simulink model "ACC_speed_change_curve_cs"  (R2016a)
settings: Solver=ode5  SolverMode=SingleTasking  StartTime=0.0  StopTime=inf  FixedStep=1/1000  RelTol=1e-3
PreLoadFcn:
  | mbxruntime.callbacks.PreLoadFcn(bdroot);
  | check_NUTS_defined;
  | 
  | assignin('base',['model_closed_' bdroot],false);addpath('../includes_ACC');
PostLoadFcn:
  | mbxruntime.callbacks.PostLoadFcn(bdroot);
InitFcn:
  | mbxruntime.callbacks.InitFcn(bdroot);
StartFcn:
  | mbxruntime.callbacks.StartFcn(bdroot);
StopFcn:
  | mbxruntime.callbacks.StopFcn(bdroot);
model workspace (MAT data in the model file):
  mbox_table : struct (value not decoded)
  model_closed = 0
  sim_status = 0
undefined symbols (not defined in the file or in its folder): DiscIntNeverNeededParam
undefined symbols (not defined in the file): SteeringColumn, SteeringWheel, WheelL0, WheelL1, WheelR0, WheelR1
libraries: simulink_extras x49, simulink x29, PreScanSimulinkLibrary x24, PreScanUsefulBlocks x2, Solver_SF x1, simulink_need_slupdate x1
(part 17 of 17)

== system ACC_speed_change_curve_cs/Audi_A8_1/ACC_System3/TIS2 ACC action/Stop & Go/Subsystem ==
  In1 : Inport
  In2 : Inport  Port=2
  EGO_Velocity [m/s] : Inport  Port=3
  Abs : Abs
  Abs1 : Abs
  Compare To Constant : simulink/Logic and Bit Operations/Compare To Constant  relop=<=  const=0.1  OutDataTypeStr=uint8  ZeroCross=off
  Compare To Constant1 : simulink/Logic and Bit Operations/Compare To Constant  relop=<=  const=0.1  OutDataTypeStr=uint8  ZeroCross=off
  Logical Operator1 : Logic  AllPortsSameDT=off  OutDataTypeStr=boolean
  Max Brake ON : Constant  Value=BrakeMax * J_xx / Qfac / Rw
  Switch1 : Switch  Criteria=u2 > Threshold
  BrakePres[bar] : Outport
  wires:
  In2/1 -> Switch1/3
  Abs1/1 -> Compare To Constant1/1
  Abs/1 -> Compare To Constant/1
  Switch1/1 -> BrakePres[bar]/1
  Max Brake ON/1 -> Switch1/1
  Logical Operator1/1 -> Switch1/2
  Compare To Constant1/1 -> Logical Operator1/2
  Compare To Constant/1 -> Logical Operator1/1
  EGO_Velocity [m/s]/1 -> Abs1/1
  In1/1 -> Abs/1

== system ACC_speed_change_curve_cs/Audi_A8_1/ACC_System3/TIS2 Bend Road/Hold/If Action Subsystem ==
  In1 : Inport
  Action Port : ActionPort  InitializeStates=reset  PropagateVarSize=During execution  ActionType=then
  Constant : Constant
  Constant1 : Constant  Value=0
  Discrete-Time Integrator : DiscreteIntegrator  gainval=100  InitialConditionSource=external  InitialConditionSetting=State (most efficient)  SampleTime=Tsensor  LimitOutput=on  UpperSaturationLimit=1  LowerSaturationLimit=0  ICPrevOutput=DiscIntNeverNeededParam  ICPrevScaledInput=DiscIntNeverNeededParam
  Gain3 : Gain  Gain=1e6  OutDataTypeStr=double
  Switch : Switch  Criteria=u2 > Threshold
  Out1 : Outport
  wires:
  Constant1/1 -> Switch/3
  Constant/1 -> Switch/1
  Switch/1 -> Discrete-Time Integrator/2
  Discrete-Time Integrator/1 -> Out1/1
  In1/1 -> Switch/2, Gain3/1
  Gain3/1 -> Discrete-Time Integrator/1

== system ACC_speed_change_curve_cs/Audi_A8_1/ACC_System3/TIS2 Bend Road/Hold/If Action Subsystem1 ==
  In1 : Inport
  Action Port : ActionPort  PropagateVarSize=During execution  ActionType=else
  Out1 : Outport
  wires:
  In1/1 -> Out1/1

== system ACC_speed_change_curve_cs/Audi_A8_1/ACC_System3/TIS2 Bend Road/TIS1 HWT Computing/If Action Subsystem ==
  Distance [m] : Inport
  Velocity [m/s] : Inport  Port=2
  Action Port : ActionPort  PropagateVarSize=During execution  ActionType=then
  Product : Product  Inputs=*/  RndMeth=Zero
  HWT [s] : Outport
  wires:
  Product/1 -> HWT [s]/1
  Velocity [m/s]/1 -> Product/2
  Distance [m]/1 -> Product/1

== system ACC_speed_change_curve_cs/Audi_A8_1/ACC_System3/TIS2 Bend Road/TIS1 HWT Computing/If Action Subsystem1 ==
  Action Port : ActionPort  PropagateVarSize=During execution  ActionType=else
  Constant : Constant  Value=inf
  Out1 : Outport  InitialOutput=0
  wires:
  Constant/1 -> Out1/1

== system ACC_speed_change_curve_cs/Audi_A8_1/ACC_System3/TIS2 Straight Road/Hold/If Action Subsystem ==
  In1 : Inport
  Action Port : ActionPort  InitializeStates=reset  PropagateVarSize=During execution  ActionType=then
  Constant : Constant
  Constant1 : Constant  Value=0
  Discrete-Time Integrator : DiscreteIntegrator  gainval=100  InitialConditionSource=external  InitialConditionSetting=State (most efficient)  SampleTime=Tsensor  LimitOutput=on  UpperSaturationLimit=1  LowerSaturationLimit=0  ICPrevOutput=DiscIntNeverNeededParam  ICPrevScaledInput=DiscIntNeverNeededParam
  Gain3 : Gain  Gain=1e6  OutDataTypeStr=double
  Switch : Switch  Criteria=u2 > Threshold
  Out1 : Outport
  wires:
  Constant1/1 -> Switch/3
  Constant/1 -> Switch/1
  Switch/1 -> Discrete-Time Integrator/2
  Discrete-Time Integrator/1 -> Out1/1
  In1/1 -> Switch/2, Gain3/1
  Gain3/1 -> Discrete-Time Integrator/1

== system ACC_speed_change_curve_cs/Audi_A8_1/ACC_System3/TIS2 Straight Road/Hold/If Action Subsystem1 ==
  In1 : Inport
  Action Port : ActionPort  PropagateVarSize=During execution  ActionType=else
  Out1 : Outport
  wires:
  In1/1 -> Out1/1

== system ACC_speed_change_curve_cs/Audi_A8_1/ACC_System3/TIS2 Straight Road/TIS2 HWT Computing/If Action Subsystem ==
  Distance [m] : Inport
  Velocity [m/s] : Inport  Port=2
  Action Port : ActionPort  PropagateVarSize=During execution  ActionType=then
  Product : Product  Inputs=*/  RndMeth=Zero
  HWT [s] : Outport
  wires:
  Product/1 -> HWT [s]/1
  Velocity [m/s]/1 -> Product/2
  Distance [m]/1 -> Product/1

== system ACC_speed_change_curve_cs/Audi_A8_1/ACC_System3/TIS2 Straight Road/TIS2 HWT Computing/If Action Subsystem1 ==
  HWT demanded [s] : Inport
  Action Port : ActionPort  PropagateVarSize=During execution  ActionType=else
  Gain : Gain  Gain=2*ones(TISdet(2),1)
  Out1 : Outport
  wires:
  HWT demanded [s]/1 -> Gain/1
  Gain/1 -> Out1/1

== system ACC_speed_change_curve_cs/Audi_A8_1/ACC_System3/TIS2 Straight Road/TIS2 HWT Computing2/If Action Subsystem ==
  Distance [m] : Inport
  Velocity [m/s] : Inport  Port=2
  Action Port : ActionPort  PropagateVarSize=During execution  ActionType=then
  Product : Product  Inputs=*/  RndMeth=Zero
  HWT [s] : Outport
  wires:
  Product/1 -> HWT [s]/1
  Velocity [m/s]/1 -> Product/2
  Distance [m]/1 -> Product/1

== system ACC_speed_change_curve_cs/Audi_A8_1/ACC_System3/TIS2 Straight Road/TIS2 HWT Computing2/If Action Subsystem1 ==
  Action Port : ActionPort  PropagateVarSize=During execution  ActionType=else
  Constant : Constant  Value=inf
  Out1 : Outport  InitialOutput=0
  wires:
  Constant/1 -> Out1/1

== system ACC_speed_change_curve_cs/Audi_A8_1/Trajectories/Traj2State1/Traj2State2/MuxState ==
  x [m] : Inport
  y [m] : Inport  Port=2
  z [m] : Inport  Port=3
  dx [m/s] : Inport  Port=4
  dy [m/s] : Inport  Port=5
  dz [m/s] : Inport  Port=6
  R [rad] : Inport  Port=7
  P [rad] : Inport  Port=8
  Y [rad] : Inport  Port=9
  Mux : Mux  Inputs=9
  state : Outport
  wires:
  z [m]/1 -> Mux/3
  y [m]/1 -> Mux/2
  x [m]/1 -> Mux/1
  Y [rad]/1 -> Mux/9
  P [rad]/1 -> Mux/8
  R [rad]/1 -> Mux/7
  dz [m/s]/1 -> Mux/6
  dy [m/s]/1 -> Mux/5
  dx [m/s]/1 -> Mux/4
  Mux/1 -> state/1

== system ACC_speed_change_curve_cs/Audi_A8_1/Trajectories/Traj2State1/Traj2State2/Traj2MuxState_Ext ==
  Traj : Inport
  Terminator{1..9} (9 alike) : Terminator
  demux : Subsystem
  x [m] : Outport
  y [m] : Outport  Port=2
  z [m] : Outport  Port=3
  dx [m/s] : Outport  Port=4
  dy [m/s] : Outport  Port=5
  dz [m/s] : Outport  Port=6
  R [rad] : Outport  Port=7
  P [rad] : Outport  Port=8
  Y [rad] : Outport  Port=9
  wires:
  demux/9(Y) -> Y [rad]/1
  demux/7(R) -> R [rad]/1
  demux/5(vely) -> dy [m/s]/1
  demux/4(velx) -> dx [m/s]/1
  demux/10(velR) -> Terminator4/1
  demux/11(velP) -> Terminator5/1
  demux/12(velY) -> Terminator1/1
  demux/13(accx) -> Terminator8/1
  demux/14(accy) -> Terminator9/1
  demux/15(accz) -> Terminator7/1
  demux/18(accY) -> Terminator2/1
  demux/16(accR) -> Terminator3/1
  demux/17(accP) -> Terminator6/1
  demux/3(z) -> z [m]/1
  Traj/1 -> demux/1(traj)
  demux/6(velz) -> dz [m/s]/1
  demux/1(x) -> x [m]/1
  demux/2(y) -> y [m]/1
  demux/8(P) -> P [rad]/1

== system ACC_speed_change_curve_cs/BMW_X5_1/Trajectories/Traj2State1/Traj2State2/MuxState ==
  x [m] : Inport
  y [m] : Inport  Port=2
  z [m] : Inport  Port=3
  dx [m/s] : Inport  Port=4
  dy [m/s] : Inport  Port=5
  dz [m/s] : Inport  Port=6
  R [rad] : Inport  Port=7
  P [rad] : Inport  Port=8
  Y [rad] : Inport  Port=9
  Mux : Mux  Inputs=9
  state : Outport
  wires:
  z [m]/1 -> Mux/3
  y [m]/1 -> Mux/2
  x [m]/1 -> Mux/1
  Y [rad]/1 -> Mux/9
  P [rad]/1 -> Mux/8
  R [rad]/1 -> Mux/7
  dz [m/s]/1 -> Mux/6
  dy [m/s]/1 -> Mux/5
  dx [m/s]/1 -> Mux/4
  Mux/1 -> state/1

== system ACC_speed_change_curve_cs/BMW_X5_1/Trajectories/Traj2State1/Traj2State2/Traj2MuxState_Ext ==
  Traj : Inport
  Terminator{1..9} (9 alike) : Terminator
  demux : Subsystem
  x [m] : Outport
  y [m] : Outport  Port=2
  z [m] : Outport  Port=3
  dx [m/s] : Outport  Port=4
  dy [m/s] : Outport  Port=5
  dz [m/s] : Outport  Port=6
  R [rad] : Outport  Port=7
  P [rad] : Outport  Port=8
  Y [rad] : Outport  Port=9
  wires:
  demux/9(Y) -> Y [rad]/1
  demux/7(R) -> R [rad]/1
  demux/5(vely) -> dy [m/s]/1
  demux/4(velx) -> dx [m/s]/1
  demux/10(velR) -> Terminator4/1
  demux/11(velP) -> Terminator5/1
  demux/12(velY) -> Terminator1/1
  demux/13(accx) -> Terminator8/1
  demux/14(accy) -> Terminator9/1
  demux/15(accz) -> Terminator7/1
  demux/18(accY) -> Terminator2/1
  demux/16(accR) -> Terminator3/1
  demux/17(accP) -> Terminator6/1
  demux/3(z) -> z [m]/1
  Traj/1 -> demux/1(traj)
  demux/6(velz) -> dz [m/s]/1
  demux/1(x) -> x [m]/1
  demux/2(y) -> y [m]/1
  demux/8(P) -> P [rad]/1

== system ACC_speed_change_curve_cs/Toyota_Previa_1/Trajectories/Traj2State1/Traj2State2/MuxState ==
  x [m] : Inport
  y [m] : Inport  Port=2
  z [m] : Inport  Port=3
  dx [m/s] : Inport  Port=4
  dy [m/s] : Inport  Port=5
  dz [m/s] : Inport  Port=6
  R [rad] : Inport  Port=7
  P [rad] : Inport  Port=8
  Y [rad] : Inport  Port=9
  Mux : Mux  Inputs=9
  state : Outport
  wires:
  z [m]/1 -> Mux/3
  y [m]/1 -> Mux/2
  x [m]/1 -> Mux/1
  Y [rad]/1 -> Mux/9
  P [rad]/1 -> Mux/8
  R [rad]/1 -> Mux/7
  dz [m/s]/1 -> Mux/6
  dy [m/s]/1 -> Mux/5
  dx [m/s]/1 -> Mux/4
  Mux/1 -> state/1

== system ACC_speed_change_curve_cs/Toyota_Previa_1/Trajectories/Traj2State1/Traj2State2/Traj2MuxState_Ext ==
  Traj : Inport
  Terminator{1..9} (9 alike) : Terminator
  demux : Subsystem
  x [m] : Outport
  y [m] : Outport  Port=2
  z [m] : Outport  Port=3
  dx [m/s] : Outport  Port=4
  dy [m/s] : Outport  Port=5
  dz [m/s] : Outport  Port=6
  R [rad] : Outport  Port=7
  P [rad] : Outport  Port=8
  Y [rad] : Outport  Port=9
  wires:
  demux/9(Y) -> Y [rad]/1
  demux/7(R) -> R [rad]/1
  demux/5(vely) -> dy [m/s]/1
  demux/4(velx) -> dx [m/s]/1
  demux/10(velR) -> Terminator4/1
  demux/11(velP) -> Terminator5/1
  demux/12(velY) -> Terminator1/1
  demux/13(accx) -> Terminator8/1
  demux/14(accy) -> Terminator9/1
  demux/15(accz) -> Terminator7/1
  demux/18(accY) -> Terminator2/1
  demux/16(accR) -> Terminator3/1
  demux/17(accP) -> Terminator6/1
  demux/3(z) -> z [m]/1
  Traj/1 -> demux/1(traj)
  demux/6(velz) -> dz [m/s]/1
  demux/1(x) -> x [m]/1
  demux/2(y) -> y [m]/1
  demux/8(P) -> P [rad]/1

== system ACC_speed_change_curve_cs/Toyota_Yaris_1/Trajectories/Traj2State1/Traj2State2/MuxState ==
  x [m] : Inport
  y [m] : Inport  Port=2
  z [m] : Inport  Port=3
  dx [m/s] : Inport  Port=4
  dy [m/s] : Inport  Port=5
  dz [m/s] : Inport  Port=6
  R [rad] : Inport  Port=7
  P [rad] : Inport  Port=8
  Y [rad] : Inport  Port=9
  Mux : Mux  Inputs=9
  state : Outport
  wires:
  z [m]/1 -> Mux/3
  y [m]/1 -> Mux/2
  x [m]/1 -> Mux/1
  Y [rad]/1 -> Mux/9
  P [rad]/1 -> Mux/8
  R [rad]/1 -> Mux/7
  dz [m/s]/1 -> Mux/6
  dy [m/s]/1 -> Mux/5
  dx [m/s]/1 -> Mux/4
  Mux/1 -> state/1

== system ACC_speed_change_curve_cs/Toyota_Yaris_1/Trajectories/Traj2State1/Traj2State2/Traj2MuxState_Ext ==
  Traj : Inport
  Terminator{1..9} (9 alike) : Terminator
  demux : Subsystem
  x [m] : Outport
  y [m] : Outport  Port=2
  z [m] : Outport  Port=3
  dx [m/s] : Outport  Port=4
  dy [m/s] : Outport  Port=5
  dz [m/s] : Outport  Port=6
  R [rad] : Outport  Port=7
  P [rad] : Outport  Port=8
  Y [rad] : Outport  Port=9
  wires:
  demux/9(Y) -> Y [rad]/1
  demux/7(R) -> R [rad]/1
  demux/5(vely) -> dy [m/s]/1
  demux/4(velx) -> dx [m/s]/1
  demux/10(velR) -> Terminator4/1
  demux/11(velP) -> Terminator5/1
  demux/12(velY) -> Terminator1/1
  demux/13(accx) -> Terminator8/1
  demux/14(accy) -> Terminator9/1
  demux/15(accz) -> Terminator7/1
  demux/18(accY) -> Terminator2/1
  demux/16(accR) -> Terminator3/1
  demux/17(accP) -> Terminator6/1
  demux/3(z) -> z [m]/1
  Traj/1 -> demux/1(traj)
  demux/6(velz) -> dz [m/s]/1
  demux/1(x) -> x [m]/1
  demux/2(y) -> y [m]/1
  demux/8(P) -> P [rad]/1

== system ACC_speed_change_curve_cs/Audi_A8_1/ACC_System3/TIS1 ACC action/If Action Subsystem/If Action Subsystem/Subsystem ==
  e : Inport
  Difference : simulink/Discrete/Difference  ICPrevInput=0.0  InputProcessing=Inherited  OutMin=[]  OutMax=[]  OutDataType=sfix(16)  OutScaling=2^-10  DoSatur=off
  Discrete-Time Integrator : DiscreteIntegrator  SampleTime=Tsensor  ICPrevOutput=DiscIntNeverNeededParam  ICPrevScaledInput=DiscIntNeverNeededParam
  Gain : Gain  Gain=100
  Gain1 : Gain  Gain=0.5
  Gain2 : Gain  Gain=3.065*0.01
  Sum : Sum  Inputs=+++
  out : Outport
  wires:
  Sum/1 -> out/1
  Difference/1 -> Sum/3
  Discrete-Time Integrator/1 -> Sum/2
  Gain/1 -> Sum/1
  Gain2/1 -> Difference/1
  Gain1/1 -> Discrete-Time Integrator/1
  e/1 -> Gain2/1, Gain/1, Gain1/1

== system ACC_speed_change_curve_cs/Audi_A8_1/ACC_System3/TIS1 ACC action/If Action Subsystem/If Action Subsystem1/If Action Subsystem ==
  rd : Inport
  e [m] : Inport  Port=2
  Action Port : ActionPort  PropagateVarSize=During execution  ActionType=then
  Abs : Abs
  Constant : Constant  Value=0
  Divide : Product  Inputs=*/
  Gain : Gain  Gain=0.5
  Math Function : Math  Operator=square  SaturateOnIntegerOverflow=on
  Saturation1 : Saturate  UpperLimit=inf  LowerLimit=0.02
  deceleration_[m/s2] : Outport  InitialOutput=0
  throttle : Outport  Port=2  InitialOutput=0
  wires:
  Constant/1 -> throttle/1
  Gain/1 -> deceleration_[m/s2]/1
  e [m]/1 -> Abs/1
  Saturation1/1 -> Divide/2
  Abs/1 -> Saturation1/1
  Math Function/1 -> Divide/1
  Divide/1 -> Gain/1
  rd/1 -> Math Function/1

== system ACC_speed_change_curve_cs/Audi_A8_1/ACC_System3/TIS1 ACC action/If Action Subsystem/If Action Subsystem1/If Action Subsystem1 ==
  rd : Inport
  e [m] : Inport  Port=2
  EGO_distance[m] : Inport  Port=3
  HWT_dem : Inport  Port=4
  Vp : Inport  Port=5
  e_acc : Inport  Port=6
  th_in : Inport  Port=7
  Action Port : ActionPort  PropagateVarSize=During execution  ActionType=else
  Add : Sum  Inputs=+-
  If : If  SampleTime=Tsensor
  If Action Subsystem : Subsystem  TreatAsAtomicUnit=on
  If Action Subsystem1 : Subsystem  TreatAsAtomicUnit=on
  Merge : Merge
  Merge1 : Merge
  Product : Product  RndMeth=Zero
  Vp1 : InportShadow  Port=5
  throttle : Outport  InitialOutput=0
  brake : Outport  Port=2  InitialOutput=0
  wires:
  th_in/1 -> If Action Subsystem/2(th_in)
  e_acc/1 -> If Action Subsystem/1(e)
  If Action Subsystem/2(throttle) -> Merge/1
  If Action Subsystem/1(brake) -> Merge1/1
  Merge/1 -> throttle/1
  Merge1/1 -> brake/1
  If Action Subsystem1/1(throttle) -> Merge/2
  If Action Subsystem1/2(brake) -> Merge1/2
  Vp/1 -> If Action Subsystem1/1(Vp)
  e [m]/1 -> If Action Subsystem1/3(e [m])
  rd/1 -> If Action Subsystem1/2(rd)
  If/2 -> If Action Subsystem1/Action
  If/1 -> If Action Subsystem/Action
  Add/1 -> If/1
  Product/1 -> Add/2
  EGO_distance[m]/1 -> Add/1
  Vp1/1 -> Product/2
  HWT_dem/1 -> Product/1

== system ACC_speed_change_curve_cs/Audi_A8_1/ACC_System3/TIS1 ACC action/If Action Subsystem1/If Action Subsystem1/If Action Subsystem ==
  Action Port : ActionPort  PropagateVarSize=During execution  ActionType=then
  Constant : Constant  Value=0
  Constant1 : Constant  Value=BrakeMax
  dec : Outport  InitialOutput=0
  throttle : Outport  Port=2  InitialOutput=0
  wires:
  Constant1/1 -> dec/1
  Constant/1 -> throttle/1

== system ACC_speed_change_curve_cs/Audi_A8_1/ACC_System3/TIS1 ACC action/If Action Subsystem1/If Action Subsystem1/If Action Subsystem1 ==
  rd : Inport
  e [m] : Inport  Port=2
  EGO_distance[m] : Inport  Port=3
  HWT_dem : Inport  Port=4
  Vp : Inport  Port=5
  Action Port : ActionPort  PropagateVarSize=During execution  ActionType=else
  Add : Sum  Inputs=+-
  If : If  SampleTime=Tsensor
  If Action Subsystem : Subsystem  TreatAsAtomicUnit=on
  If Action Subsystem1 : Subsystem  TreatAsAtomicUnit=on
  Merge : Merge
  Merge1 : Merge
  Product : Product  RndMeth=Zero
  Vp1 : InportShadow  Port=5
  throttle : Outport  InitialOutput=0
  brake : Outport  Port=2  InitialOutput=0
  wires:
  If Action Subsystem1/1(throttle) -> Merge/2
  If Action Subsystem1/2(brake) -> Merge1/2
  If Action Subsystem/2(throttle) -> Merge/1
  If Action Subsystem/1(brake) -> Merge1/1
  Merge/1 -> throttle/1
  Merge1/1 -> brake/1
  Vp/1 -> If Action Subsystem1/1(Vp)
  e [m]/1 -> If Action Subsystem1/3(e [m])
  rd/1 -> If Action Subsystem1/2(rd)
  If/2 -> If Action Subsystem1/Action
  If/1 -> If Action Subsystem/Action
  Add/1 -> If/1
  Product/1 -> Add/2
  EGO_distance[m]/1 -> Add/1
  Vp1/1 -> Product/2
  HWT_dem/1 -> Product/1

== system ACC_speed_change_curve_cs/Audi_A8_1/ACC_System3/TIS2 ACC action/If Action Subsystem/If Action Subsystem/Subsystem ==
  e : Inport
  Constant : Constant  Value=p
  Constant1 : Constant  Value=i
  Constant2 : Constant  Value=d
  Difference : simulink/Discrete/Difference  ICPrevInput=0.0  InputProcessing=Inherited  OutMin=[]  OutMax=[]  OutDataType=sfix(16)  OutScaling=2^-10  DoSatur=off
  Discrete-Time Integrator : DiscreteIntegrator  SampleTime=-1  ICPrevOutput=DiscIntNeverNeededParam  ICPrevScaledInput=DiscIntNeverNeededParam
  Gain1 : Gain  Gain=0.3
  Gain2 : Gain  Gain=3.065*0.01
  Product : Product
  Product1 : Product
  Product2 : Product
  Sum : Sum  Inputs=+++
  out : Outport
  wires:
  Sum/1 -> out/1
  Difference/1 -> Sum/3
  Discrete-Time Integrator/1 -> Sum/2
  Product/1 -> Sum/1
  Product2/1 -> Difference/1
  Product1/1 -> Discrete-Time Integrator/1
  e/1 -> Product1/2, Product/2, Product2/1
  Constant/1 -> Product/1
  Constant1/1 -> Product1/1
  Constant2/1 -> Product2/2

== system ACC_speed_change_curve_cs/Audi_A8_1/ACC_System3/TIS2 ACC action/If Action Subsystem/If Action Subsystem1/If Action Subsystem ==
  rd : Inport
  e [m] : Inport  Port=2
  Action Port : ActionPort  PropagateVarSize=During execution  ActionType=then
  Abs : Abs
  Constant : Constant  Value=0
  Constant1 : Constant  Value=b
  Divide : Product  Inputs=*/
  Gain : Gain  Gain=0.5
  Math Function : Math  Operator=square  SaturateOnIntegerOverflow=on
  Product : Product
  Saturation1 : Saturate  UpperLimit=inf  LowerLimit=0.02
  deceleration_[m/s2] : Outport  InitialOutput=0
  throttle : Outport  Port=2  InitialOutput=0
  wires:
  Constant/1 -> throttle/1
  Product/1 -> deceleration_[m/s2]/1
  e [m]/1 -> Abs/1
  Saturation1/1 -> Divide/2
  Abs/1 -> Saturation1/1
  Math Function/1 -> Divide/1
  Divide/1 -> Product/2
  rd/1 -> Math Function/1
  Constant1/1 -> Product/1

== system ACC_speed_change_curve_cs/Audi_A8_1/ACC_System3/TIS2 ACC action/If Action Subsystem/If Action Subsystem1/If Action Subsystem1 ==
  rd : Inport
  e [m] : Inport  Port=2
  EGO_distance[m] : Inport  Port=3
  HWT_dem : Inport  Port=4
  Vp : Inport  Port=5
  e_acc : Inport  Port=6
  th_in : Inport  Port=7
  Action Port : ActionPort  PropagateVarSize=During execution  ActionType=else
  Add : Sum  Inputs=+-
  If : If
  If Action Subsystem : Subsystem  TreatAsAtomicUnit=on
  If Action Subsystem1 : Subsystem  TreatAsAtomicUnit=on
  Merge : Merge
  Merge1 : Merge
  Product : Product  RndMeth=Zero
  Vp1 : InportShadow  Port=5
  throttle : Outport  InitialOutput=0
  brake : Outport  Port=2  InitialOutput=0
  wires:
  th_in/1 -> If Action Subsystem/2(th_in)
  e_acc/1 -> If Action Subsystem/1(e)
  If Action Subsystem/2(throttle) -> Merge/1
  If Action Subsystem/1(brake) -> Merge1/1
  Merge/1 -> throttle/1
  Merge1/1 -> brake/1
  If Action Subsystem1/1(throttle) -> Merge/2
  If Action Subsystem1/2(brake) -> Merge1/2
  Vp/1 -> If Action Subsystem1/1(Vp)
  e [m]/1 -> If Action Subsystem1/3(e [m])
  rd/1 -> If Action Subsystem1/2(rd)
  If/2 -> If Action Subsystem1/Action
  If/1 -> If Action Subsystem/Action
  Add/1 -> If/1
  Product/1 -> Add/2
  EGO_distance[m]/1 -> Add/1
  Vp1/1 -> Product/2
  HWT_dem/1 -> Product/1

== system ACC_speed_change_curve_cs/Audi_A8_1/ACC_System3/TIS2 ACC action/If Action Subsystem1/If Action Subsystem1/If Action Subsystem ==
  Action Port : ActionPort  PropagateVarSize=During execution  ActionType=then
  Constant : Constant  Value=0
  Constant1 : Constant  Value=BrakeMax
  dec : Outport  InitialOutput=0
  throttle : Outport  Port=2  InitialOutput=0
  wires:
  Constant1/1 -> dec/1
  Constant/1 -> throttle/1

== system ACC_speed_change_curve_cs/Audi_A8_1/ACC_System3/TIS2 ACC action/If Action Subsystem1/If Action Subsystem1/If Action Subsystem1 ==
  rd : Inport
  e [m] : Inport  Port=2
  EGO_distance[m] : Inport  Port=3
  HWT_dem : Inport  Port=4
  Vp : Inport  Port=5
  Action Port : ActionPort  PropagateVarSize=During execution  ActionType=else
  Add : Sum  Inputs=+-
  If : If
  If Action Subsystem : Subsystem  TreatAsAtomicUnit=on
  If Action Subsystem1 : Subsystem  TreatAsAtomicUnit=on
  Merge : Merge
  Merge1 : Merge
  Product : Product  RndMeth=Zero
  Vp1 : InportShadow  Port=5
  throttle : Outport  InitialOutput=0
  brake : Outport  Port=2  InitialOutput=0
  wires:
  If Action Subsystem/2(throttle) -> Merge/1
  If Action Subsystem/1(brake) -> Merge1/1
  Merge/1 -> throttle/1
  Merge1/1 -> brake/1
  If Action Subsystem1/1(throttle) -> Merge/2
  If Action Subsystem1/2(brake) -> Merge1/2
  Vp/1 -> If Action Subsystem1/1(Vp)
  e [m]/1 -> If Action Subsystem1/3(e [m])
  rd/1 -> If Action Subsystem1/2(rd)
  If/2 -> If Action Subsystem1/Action
  If/1 -> If Action Subsystem/Action
  Add/1 -> If/1
  Product/1 -> Add/2
  EGO_distance[m]/1 -> Add/1
  Vp1/1 -> Product/2
  HWT_dem/1 -> Product/1

== system ACC_speed_change_curve_cs/Audi_A8_1/ACC_System3/TIS2 ACC action/Stop & Go/If Action Subsystem/If Action Subsystem ==
  rd : Inport
  e [m] : Inport  Port=2
  th_in : Inport  Port=3
  dis : Inport  Port=4
  Stand : Inport  Port=5
  Action Port : ActionPort  PropagateVarSize=During execution  ActionType=then
  If : If
  If Action Subsystem : Subsystem  TreatAsAtomicUnit=on
  If Action Subsystem1 : Subsystem  TreatAsAtomicUnit=on
  Merge : Merge
  Merge1 : Merge
  brake : Outport  InitialOutput=0
  throttle : Outport  Port=2  InitialOutput=0
  wires:
  Stand/1 -> If Action Subsystem/4(stand)
  dis/1 -> If Action Subsystem/3(dis)
  th_in/1 -> If Action Subsystem1/2(th_in)
  If Action Subsystem1/2(throttle) -> Merge1/2
  If Action Subsystem1/1(brake) -> Merge/2
  Merge/1 -> brake/1
  Merge1/1 -> throttle/1
  If Action Subsystem/2(throttle) -> Merge1/1
  If Action Subsystem/1(brake) -> Merge/1
  If/2 -> If Action Subsystem1/Action
  e [m]/1 -> If Action Subsystem1/1(e), If Action Subsystem/2(e [m])
  If/1 -> If Action Subsystem/Action
  rd/1 -> If Action Subsystem/1(rd), If/1

== system ACC_speed_change_curve_cs/Audi_A8_1/ACC_System3/TIS2 ACC action/Stop & Go/If Action Subsystem/If Action Subsystem1 ==
  rd1 : Inport
  e [m] : Inport  Port=2
  Vp : Inport  Port=3
  dis : Inport  Port=4
  stand : Inport  Port=5
  Action Port : ActionPort  PropagateVarSize=During execution  ActionType=else
  Abs : Abs
  Add : Sum  Inputs=+-
  Bias : Bias  Bias=1
  Constant : Constant  Value=0
  Constant1 : Constant  Value=0
  Constant2 : Constant  Value=BrakeMax*J_xx/Qfac/Rw
  Constant3 : Constant  Value=BrakeMax*J_xx/Qfac/Rw
  Divide : Product  Inputs=*/
  Gain : Gain  Gain=0.5
  Gain1 : Gain  Gain=J_xx/Qfac/Rw
  Math Function : Math  Operator=square  SaturateOnIntegerOverflow=on
  Saturation : Saturate  UpperLimit=BrakeMax  LowerLimit=0
  Saturation1 : Saturate  UpperLimit=inf  LowerLimit=0.02
  Switch : Switch  Criteria=u2 > Threshold
  Switch1 : Switch  Criteria=u2 > Threshold  Threshold=1
  Switch2 : Switch  Criteria=u2 > Threshold
  rd2 : InportShadow
  brake : Outport  InitialOutput=0
  throttle1 : Outport  Port=2  InitialOutput=0
  wires:
  Switch1/1 -> Switch2/1
  Switch2/1 -> brake/1
  Bias/1 -> Add/1
  Constant3/1 -> Switch2/3
  Add/1 -> Switch2/2
  stand/1 -> Add/2
  dis/1 -> Bias/1
  Constant2/1 -> Switch1/3
  Switch/1 -> Switch1/1
  Vp/1 -> Switch1/2
  Constant1/1 -> Switch/3
  Gain1/1 -> Switch/1
  rd2/1 -> Switch/2
  Gain/1 -> Saturation/1
  Saturation/1 -> Gain1/1
  Constant/1 -> throttle1/1
  e [m]/1 -> Abs/1
  Saturation1/1 -> Divide/2
  Abs/1 -> Saturation1/1
  Math Function/1 -> Divide/1
  Divide/1 -> Gain/1
  rd1/1 -> Math Function/1

== system ACC_speed_change_curve_cs/Audi_A8_1/Trajectories/Traj2State1/Traj2State2/Traj2MuxState_Ext/demux ==
  traj : Inport
  Demux : Demux  Outputs=18
  x : Outport
  y : Outport  Port=2
  z : Outport  Port=3
  velx : Outport  Port=4
  vely : Outport  Port=5
  velz : Outport  Port=6
  R : Outport  Port=7
  P : Outport  Port=8
  Y : Outport  Port=9
  velR : Outport  Port=10
  velP : Outport  Port=11
  velY : Outport  Port=12
  accx : Outport  Port=13
  accy : Outport  Port=14
  accz : Outport  Port=15
  accR : Outport  Port=16
  accP : Outport  Port=17
  accY : Outport  Port=18
  wires:
  Demux/18 -> accY/1
  Demux/17 -> accP/1
  Demux/16 -> accR/1
  Demux/15 -> accz/1
  Demux/14 -> accy/1
  Demux/13 -> accx/1
  Demux/12 -> velY/1
  Demux/11 -> velP/1
  Demux/10 -> velR/1
  Demux/9 -> velz/1
  Demux/8 -> vely/1
  Demux/7 -> velx/1
  Demux/6 -> Y/1
  Demux/5 -> P/1
  traj/1 -> Demux/1
  Demux/4 -> R/1
  Demux/3 -> z/1
  Demux/2 -> y/1
  Demux/1 -> x/1

== system ACC_speed_change_curve_cs/BMW_X5_1/Trajectories/Traj2State1/Traj2State2/Traj2MuxState_Ext/demux ==
  traj : Inport
  Demux : Demux  Outputs=18
  x : Outport
  y : Outport  Port=2
  z : Outport  Port=3
  velx : Outport  Port=4
  vely : Outport  Port=5
  velz : Outport  Port=6
  R : Outport  Port=7
  P : Outport  Port=8
  Y : Outport  Port=9
  velR : Outport  Port=10
  velP : Outport  Port=11
  velY : Outport  Port=12
  accx : Outport  Port=13
  accy : Outport  Port=14
  accz : Outport  Port=15
  accR : Outport  Port=16
  accP : Outport  Port=17
  accY : Outport  Port=18
  wires:
  Demux/18 -> accY/1
  Demux/17 -> accP/1
  Demux/16 -> accR/1
  Demux/15 -> accz/1
  Demux/14 -> accy/1
  Demux/13 -> accx/1
  Demux/12 -> velY/1
  Demux/11 -> velP/1
  Demux/10 -> velR/1
  Demux/9 -> velz/1
  Demux/8 -> vely/1
  Demux/7 -> velx/1
  Demux/6 -> Y/1
  Demux/5 -> P/1
  traj/1 -> Demux/1
  Demux/4 -> R/1
  Demux/3 -> z/1
  Demux/2 -> y/1
  Demux/1 -> x/1

== system ACC_speed_change_curve_cs/Toyota_Previa_1/Trajectories/Traj2State1/Traj2State2/Traj2MuxState_Ext/demux ==
  traj : Inport
  Demux : Demux  Outputs=18
  x : Outport
  y : Outport  Port=2
  z : Outport  Port=3
  velx : Outport  Port=4
  vely : Outport  Port=5
  velz : Outport  Port=6
  R : Outport  Port=7
  P : Outport  Port=8
  Y : Outport  Port=9
  velR : Outport  Port=10
  velP : Outport  Port=11
  velY : Outport  Port=12
  accx : Outport  Port=13
  accy : Outport  Port=14
  accz : Outport  Port=15
  accR : Outport  Port=16
  accP : Outport  Port=17
  accY : Outport  Port=18
  wires:
  Demux/18 -> accY/1
  Demux/17 -> accP/1
  Demux/16 -> accR/1
  Demux/15 -> accz/1
  Demux/14 -> accy/1
  Demux/13 -> accx/1
  Demux/12 -> velY/1
  Demux/11 -> velP/1
  Demux/10 -> velR/1
  Demux/9 -> velz/1
  Demux/8 -> vely/1
  Demux/7 -> velx/1
  Demux/6 -> Y/1
  Demux/5 -> P/1
  traj/1 -> Demux/1
  Demux/4 -> R/1
  Demux/3 -> z/1
  Demux/2 -> y/1
  Demux/1 -> x/1

== system ACC_speed_change_curve_cs/Toyota_Yaris_1/Trajectories/Traj2State1/Traj2State2/Traj2MuxState_Ext/demux ==
  traj : Inport
  Demux : Demux  Outputs=18
  x : Outport
  y : Outport  Port=2
  z : Outport  Port=3
  velx : Outport  Port=4
  vely : Outport  Port=5
  velz : Outport  Port=6
  R : Outport  Port=7
  P : Outport  Port=8
  Y : Outport  Port=9
  velR : Outport  Port=10
  velP : Outport  Port=11
  velY : Outport  Port=12
  accx : Outport  Port=13
  accy : Outport  Port=14
  accz : Outport  Port=15
  accR : Outport  Port=16
  accP : Outport  Port=17
  accY : Outport  Port=18
  wires:
  Demux/18 -> accY/1
  Demux/17 -> accP/1
  Demux/16 -> accR/1
  Demux/15 -> accz/1
  Demux/14 -> accy/1
  Demux/13 -> accx/1
  Demux/12 -> velY/1
  Demux/11 -> velP/1
  Demux/10 -> velR/1
  Demux/9 -> velz/1
  Demux/8 -> vely/1
  Demux/7 -> velx/1
  Demux/6 -> Y/1
  Demux/5 -> P/1
  traj/1 -> Demux/1
  Demux/4 -> R/1
  Demux/3 -> z/1
  Demux/2 -> y/1
  Demux/1 -> x/1

== system ACC_speed_change_curve_cs/Audi_A8_1/ACC_System3/TIS1 ACC action/If Action Subsystem/If Action Subsystem1/If Action Subsystem1/If Action Subsystem ==
  e : Inport
  th_in : Inport  Port=2
  Action Port : ActionPort  PropagateVarSize=During execution  ActionType=then
  Constant : Constant  Value=0
  Constant1 : Constant  Value=0
  Rate Limiter : RateLimiter  RisingSlewLimit=BrakeMax*1e3  FallingSlewLimit=-BrakeMax*1e3  SampleTimeMode=inherited
  Saturation Dynamic : simulink/Discontinuities/Saturation Dynamic  OutMin=[]  OutMax=[]  OutDataTypeStr=Inherit: Same as second input  OutDataType=fixdt(1, 16)  OutScaling=2^-10  DoSatur=off
  Subsystem : Subsystem
  brake : Outport  InitialOutput=0
  throttle : Outport  Port=2  InitialOutput=0
  wires:
  Constant1/1 -> Saturation Dynamic/3
  th_in/1 -> Saturation Dynamic/1
  Rate Limiter/1 -> throttle/1
  Constant/1 -> brake/1
  Saturation Dynamic/1 -> Rate Limiter/1
  e/1 -> Subsystem/1(e)
  Subsystem/1(out) -> Saturation Dynamic/2

== system ACC_speed_change_curve_cs/Audi_A8_1/ACC_System3/TIS1 ACC action/If Action Subsystem/If Action Subsystem1/If Action Subsystem1/If Action Subsystem1 ==
  Vp : Inport
  rd : Inport  Port=2
  e [m] : Inport  Port=3
  Action Port : ActionPort  PropagateVarSize=During execution  ActionType=else
  Abs : Abs
  Constant1 : Constant  Value=0
  Constant2 : Constant  Value=LowSpeedActv
  Constant3 : Constant  Value=0
  Divide : Product  Inputs=*/
  Gain : Gain  Gain=3.6
  Gain1 : Gain  Gain=0.5
  Math Function : Math  Operator=square  SaturateOnIntegerOverflow=on
  Relational Operator : RelationalOperator  Operator=<  OutDataTypeStr=boolean
  Saturation1 : Saturate  UpperLimit=inf  LowerLimit=0.02
  Switch : Switch  Criteria=u2 > Threshold
  throttle : Outport  InitialOutput=0
  brake : Outport  Port=2  InitialOutput=0
  wires:
  Switch/1 -> brake/1
  e [m]/1 -> Abs/1
  Saturation1/1 -> Divide/2
  Abs/1 -> Saturation1/1
  Math Function/1 -> Divide/1
  Divide/1 -> Gain1/1
  rd/1 -> Math Function/1
  Constant3/1 -> Switch/3
  Gain1/1 -> Switch/1
  Relational Operator/1 -> Switch/2
  Constant2/1 -> Relational Operator/2
  Gain/1 -> Relational Operator/1
  Vp/1 -> Gain/1
  Constant1/1 -> throttle/1

== system ACC_speed_change_curve_cs/Audi_A8_1/ACC_System3/TIS1 ACC action/If Action Subsystem1/If Action Subsystem1/If Action Subsystem1/If Action Subsystem ==
  Action Port : ActionPort  PropagateVarSize=During execution  ActionType=then
  Constant : Constant  Value=0
  Constant1 : Constant  Value=0
  brake : Outport  InitialOutput=0
  throttle : Outport  Port=2  InitialOutput=0
  wires:
  Constant1/1 -> throttle/1
  Constant/1 -> brake/1

== system ACC_speed_change_curve_cs/Audi_A8_1/ACC_System3/TIS1 ACC action/If Action Subsystem1/If Action Subsystem1/If Action Subsystem1/If Action Subsystem1 ==
  Vp : Inport
  rd : Inport  Port=2
  e [m] : Inport  Port=3
  Action Port : ActionPort  PropagateVarSize=During execution  ActionType=else
  Abs : Abs
  Constant1 : Constant  Value=0
  Constant2 : Constant  Value=LowSpeedActv
  Constant3 : Constant  Value=0
  Divide : Product  Inputs=*/
  Gain : Gain  Gain=3.6
  Gain1 : Gain  Gain=0.5
  Math Function : Math  Operator=square  SaturateOnIntegerOverflow=on
  Relational Operator : RelationalOperator  Operator=<  OutDataTypeStr=boolean
  Saturation1 : Saturate  UpperLimit=inf  LowerLimit=0.02
  Switch : Switch  Criteria=u2 > Threshold
  throttle : Outport  InitialOutput=0
  brake : Outport  Port=2  InitialOutput=0
  wires:
  Switch/1 -> brake/1
  e [m]/1 -> Abs/1
  Saturation1/1 -> Divide/2
  Abs/1 -> Saturation1/1
  Math Function/1 -> Divide/1
  Divide/1 -> Gain1/1
  rd/1 -> Math Function/1
  Constant3/1 -> Switch/3
  Gain1/1 -> Switch/1
  Relational Operator/1 -> Switch/2
  Constant2/1 -> Relational Operator/2
  Gain/1 -> Relational Operator/1
  Vp/1 -> Gain/1
  Constant1/1 -> throttle/1

== system ACC_speed_change_curve_cs/Audi_A8_1/ACC_System3/TIS2 ACC action/If Action Subsystem/If Action Subsystem1/If Action Subsystem1/If Action Subsystem ==
  e : Inport
  th_in : Inport  Port=2
  Action Port : ActionPort  PropagateVarSize=During execution  ActionType=then
  Constant : Constant  Value=0
  Constant1 : Constant  Value=0
  Rate Limiter : RateLimiter  RisingSlewLimit=BrakeRateMax  FallingSlewLimit=-BrakeRateMax  SampleTimeMode=inherited
  Saturation Dynamic : simulink/Discontinuities/Saturation Dynamic  OutMin=[]  OutMax=[]  OutDataTypeStr=Inherit: Same as second input  OutDataType=fixdt(1, 16)  OutScaling=2^-10  DoSatur=off
  Subsystem : Subsystem
  brake : Outport  InitialOutput=0
  throttle : Outport  Port=2  InitialOutput=0
  wires:
  Constant1/1 -> Saturation Dynamic/3
  th_in/1 -> Saturation Dynamic/1
  Rate Limiter/1 -> throttle/1
  Constant/1 -> brake/1
  Saturation Dynamic/1 -> Rate Limiter/1
  e/1 -> Subsystem/1(e)
  Subsystem/1(out) -> Saturation Dynamic/2

== system ACC_speed_change_curve_cs/Audi_A8_1/ACC_System3/TIS2 ACC action/If Action Subsystem/If Action Subsystem1/If Action Subsystem1/If Action Subsystem1 ==
  Vp : Inport
  rd : Inport  Port=2
  e [m] : Inport  Port=3
  Action Port : ActionPort  PropagateVarSize=During execution  ActionType=else
  Abs : Abs
  Constant1 : Constant  Value=0
  Constant2 : Constant  Value=LowSpeedActv
  Constant3 : Constant  Value=0
  Constant4 : Constant  Value=b
  Divide : Product  Inputs=*/
  Gain : Gain  Gain=3.6
  Math Function : Math  Operator=square  SaturateOnIntegerOverflow=on
  Product : Product
  Relational Operator : RelationalOperator  Operator=<  OutDataTypeStr=boolean
  Saturation1 : Saturate  UpperLimit=inf  LowerLimit=0.02
  Switch : Switch  Criteria=u2 > Threshold
  throttle : Outport  InitialOutput=0
  brake : Outport  Port=2  InitialOutput=0
  wires:
  Switch/1 -> brake/1
  e [m]/1 -> Abs/1
  Saturation1/1 -> Divide/2
  Abs/1 -> Saturation1/1
  Math Function/1 -> Divide/1
  rd/1 -> Math Function/1
  Constant3/1 -> Switch/3
  Product/1 -> Switch/1
  Relational Operator/1 -> Switch/2
  Constant2/1 -> Relational Operator/2
  Gain/1 -> Relational Operator/1
  Vp/1 -> Gain/1
  Constant1/1 -> throttle/1
  Divide/1 -> Product/2
  Constant4/1 -> Product/1

== system ACC_speed_change_curve_cs/Audi_A8_1/ACC_System3/TIS2 ACC action/If Action Subsystem1/If Action Subsystem1/If Action Subsystem1/If Action Subsystem ==
  Action Port : ActionPort  PropagateVarSize=During execution  ActionType=then
  Constant : Constant  Value=0
  Constant1 : Constant  Value=0
  brake : Outport  InitialOutput=0
  throttle : Outport  Port=2  InitialOutput=0
  wires:
  Constant1/1 -> throttle/1
  Constant/1 -> brake/1

== system ACC_speed_change_curve_cs/Audi_A8_1/ACC_System3/TIS2 ACC action/If Action Subsystem1/If Action Subsystem1/If Action Subsystem1/If Action Subsystem1 ==
  Vp : Inport
  rd : Inport  Port=2
  e [m] : Inport  Port=3
  Action Port : ActionPort  PropagateVarSize=During execution  ActionType=else
  Abs : Abs
  Constant1 : Constant  Value=0
  Constant2 : Constant  Value=LowSpeedActv
  Constant3 : Constant  Value=0
  Constant4 : Constant  Value=b
  Divide : Product  Inputs=*/
  Gain : Gain  Gain=3.6
  Gain1 : Gain  Gain=0.5
  Math Function : Math  Operator=square  SaturateOnIntegerOverflow=on
  Product : Product
  Relational Operator : RelationalOperator  Operator=<  OutDataTypeStr=boolean
  Saturation1 : Saturate  UpperLimit=inf  LowerLimit=0.02
  Switch : Switch  Criteria=u2 > Threshold
  throttle : Outport  InitialOutput=0
  brake : Outport  Port=2  InitialOutput=0
  wires:
  Switch/1 -> brake/1
  e [m]/1 -> Abs/1
  Saturation1/1 -> Divide/2
  Abs/1 -> Saturation1/1
  Math Function/1 -> Divide/1
  Divide/1 -> Product/2
  rd/1 -> Math Function/1
  Constant3/1 -> Switch/3
  Product/1 -> Switch/1
  Relational Operator/1 -> Switch/2
  Constant2/1 -> Relational Operator/2
  Gain/1 -> Relational Operator/1
  Vp/1 -> Gain/1
  Constant1/1 -> throttle/1
  Constant4/1 -> Product/1

== system ACC_speed_change_curve_cs/Audi_A8_1/ACC_System3/TIS2 ACC action/Stop & Go/If Action Subsystem/If Action Subsystem/If Action Subsystem ==
  rd : Inport
  e [m] : Inport  Port=2
  dis : Inport  Port=3
  stand : Inport  Port=4
  Action Port : ActionPort  PropagateVarSize=During execution  ActionType=then
  Abs : Abs
  Add : Sum  Inputs=+-
  Bias : Bias  Bias=1
  Constant : Constant  Value=0
  Constant1 : Constant  Value=BrakeMax
  Divide : Product  Inputs=*/
  Gain : Gain  Gain=0.5
  Gain1 : Gain  Gain=J_xx/Qfac/Rw
  Math Function : Math  Operator=square  SaturateOnIntegerOverflow=on
  Saturation : Saturate  UpperLimit=BrakeMax  LowerLimit=0
  Saturation1 : Saturate  UpperLimit=inf  LowerLimit=0.02
  Switch : Switch  Criteria=u2 > Threshold
  brake : Outport  InitialOutput=0
  throttle : Outport  Port=2  InitialOutput=0
  wires:
  Bias/1 -> Add/1
  Constant1/1 -> Switch/3
  Saturation/1 -> Switch/1
  Add/1 -> Switch/2
  stand/1 -> Add/2
  dis/1 -> Bias/1
  Switch/1 -> Gain1/1
  Gain1/1 -> brake/1
  Gain/1 -> Saturation/1
  Constant/1 -> throttle/1
  e [m]/1 -> Abs/1
  Saturation1/1 -> Divide/2
  Abs/1 -> Saturation1/1
  Math Function/1 -> Divide/1
  Divide/1 -> Gain/1
  rd/1 -> Math Function/1

== system ACC_speed_change_curve_cs/Audi_A8_1/ACC_System3/TIS2 ACC action/Stop & Go/If Action Subsystem/If Action Subsystem/If Action Subsystem1 ==
  e : Inport
  th_in : Inport  Port=2
  Action Port : ActionPort  PropagateVarSize=During execution  ActionType=else
  Constant : Constant  Value=0
  Constant1 : Constant  Value=0
  Rate Limiter : RateLimiter  RisingSlewLimit=BrakeRateMax  FallingSlewLimit=-BrakeRateMax  SampleTimeMode=inherited
  Saturation Dynamic : simulink/Discontinuities/Saturation Dynamic  OutMin=[]  OutMax=[]  OutDataTypeStr=Inherit: Same as second input  OutDataType=fixdt(1, 16)  OutScaling=2^-10  DoSatur=off
  Subsystem : Subsystem
  brake : Outport  InitialOutput=0
  throttle : Outport  Port=2  InitialOutput=0
  wires:
  Constant1/1 -> Saturation Dynamic/3
  th_in/1 -> Saturation Dynamic/1
  Rate Limiter/1 -> throttle/1
  Constant/1 -> brake/1
  Saturation Dynamic/1 -> Rate Limiter/1
  e/1 -> Subsystem/1(e)
  Subsystem/1(out) -> Saturation Dynamic/2

== system ACC_speed_change_curve_cs/Audi_A8_1/ACC_System3/TIS1 ACC action/If Action Subsystem/If Action Subsystem1/If Action Subsystem1/If Action Subsystem/Subsystem ==
  e : Inport
  Difference : simulink/Discrete/Difference  ICPrevInput=0.0  InputProcessing=Inherited  OutMin=[]  OutMax=[]  OutDataType=sfix(16)  OutScaling=2^-10  DoSatur=off
  Discrete-Time Integrator : DiscreteIntegrator  SampleTime=-1  ICPrevOutput=DiscIntNeverNeededParam  ICPrevScaledInput=DiscIntNeverNeededParam
  Gain : Gain  Gain=100
  Gain1 : Gain  Gain=0.3
  Gain2 : Gain  Gain=3.065*0.01
  Sum : Sum  Inputs=+++
  out : Outport
  wires:
  Sum/1 -> out/1
  Difference/1 -> Sum/3
  Discrete-Time Integrator/1 -> Sum/2
  Gain/1 -> Sum/1
  Gain2/1 -> Difference/1
  Gain1/1 -> Discrete-Time Integrator/1
  e/1 -> Gain2/1, Gain/1, Gain1/1

== system ACC_speed_change_curve_cs/Audi_A8_1/ACC_System3/TIS2 ACC action/If Action Subsystem/If Action Subsystem1/If Action Subsystem1/If Action Subsystem/Subsystem ==
  e : Inport
  Constant : Constant  Value=p
  Constant1 : Constant  Value=i
  Constant2 : Constant  Value=d
  Difference : simulink/Discrete/Difference  ICPrevInput=0.0  InputProcessing=Inherited  OutMin=[]  OutMax=[]  OutDataType=sfix(16)  OutScaling=2^-10  DoSatur=off
  Discrete-Time Integrator : DiscreteIntegrator  SampleTime=-1  ICPrevOutput=DiscIntNeverNeededParam  ICPrevScaledInput=DiscIntNeverNeededParam
  Product : Product
  Product1 : Product
  Product2 : Product
  Sum : Sum  Inputs=+++
  out : Outport
  wires:
  Sum/1 -> out/1
  Difference/1 -> Sum/3
  Discrete-Time Integrator/1 -> Sum/2
  Product/1 -> Sum/1
  Product2/1 -> Difference/1
  Product1/1 -> Discrete-Time Integrator/1
  e/1 -> Product/2, Product1/2, Product2/1
  Constant/1 -> Product/1
  Constant1/1 -> Product1/1
  Constant2/1 -> Product2/2

== system ACC_speed_change_curve_cs/Audi_A8_1/ACC_System3/TIS2 ACC action/Stop & Go/If Action Subsystem/If Action Subsystem/If Action Subsystem1/Subsystem ==
  e : Inport
  Difference : simulink/Discrete/Difference  ICPrevInput=0.0  InputProcessing=Inherited  OutMin=[]  OutMax=[]  OutDataType=sfix(16)  OutScaling=2^-10  DoSatur=off
  Discrete-Time Integrator : DiscreteIntegrator  SampleTime=-1  ICPrevOutput=DiscIntNeverNeededParam  ICPrevScaledInput=DiscIntNeverNeededParam
  Gain : Gain  Gain=20
  Gain1 : Gain  Gain=0.3
  Gain2 : Gain  Gain=3.065*0.01
  Sum : Sum  Inputs=+++
  out : Outport
  wires:
  Sum/1 -> out/1
  Difference/1 -> Sum/3
  Discrete-Time Integrator/1 -> Sum/2
  Gain/1 -> Sum/1
  Gain2/1 -> Difference/1
  Gain1/1 -> Discrete-Time Integrator/1
  e/1 -> Gain2/1, Gain/1, Gain1/1

== matlab function ACC_speed_change_curve_cs/Audi_A8_1/ACC_System/MATLAB Function ==
  data: distance input; simStopFlag output
function simStopFlag = distance_monitor(distance)
coder.extrinsic('set_param')
simStopFlag = 0;
if distance < 0.1
    set_param('STUDY','SimulationCommand','stop')
    simStopFlag = 1;
end
end

== matlab function ACC_speed_change_curve_cs/Audi_A8_1/ACC_System/TIS1 Bend Road/Embedded MATLAB Function ==
  data: TISMaxRange parameter; index output; distance input; TISdet parameter
function index = clsst_bjct(TISMaxRange, distance, TISdet)
% which object is the closest?

[mini, index] = min(distance);
if mini == TISMaxRange(1)
    index = TISdet(1);
end
end

== matlab function ACC_speed_change_curve_cs/Audi_A8_1/ACC_System/TIS2 Bend Road/TIS2_closest_object_search1 ==
  data: TISMaxRange parameter; distance input; index output; TISdet parameter
function index = clsst_bjct(TISMaxRange, distance, TISdet)
% which object is the closest?

[mini, index] = min(distance);
if mini == 5*TISMaxRange(2)
    index = TISdet(2);
end
end

== matlab function ACC_speed_change_curve_cs/Audi_A8_1/ACC_System/TIS1 Straight Road/TIS1_closest_object_search ==
  data: distance input; index output; TISMaxRange parameter; TISdet parameter
function index = clsst_bjct(distance, TISMaxRange, TISdet)
% which object is the closest?

[mini, index] = min(distance);
if mini == TISMaxRange(1)
    index = TISdet(1);
end

end

== matlab function ACC_speed_change_curve_cs/Audi_A8_1/ACC_System/TIS2 Straight Road/TIS2_closest_object_search ==
  data: distance input; index output; TISMaxRange parameter; TISdet parameter
function index = clsst_bjct(distance, TISMaxRange, TISdet)
% which object is the closest?

[mini, index] = min(distance);
if mini == 5*TISMaxRange(2)
    index = TISdet(2);
end
end

== matlab function ACC_speed_change_curve_cs/Audi_A8_1/ACC_System3/TIS1 Bend Road/Embedded MATLAB Function ==
  data: TISMaxRange parameter; index output; distance input; TISdet parameter
function index = clsst_bjct(TISMaxRange, distance, TISdet)
% which object is the closest?

[mini, index] = min(distance);
if mini == TISMaxRange(1)
    index = TISdet(1);
end
end

== matlab function ACC_speed_change_curve_cs/Audi_A8_1/ACC_System3/TIS1 Straight Road/TIS1_closest_object_search ==
  data: distance input; index output; TISMaxRange parameter; TISdet parameter
function index = clsst_bjct(distance, TISMaxRange, TISdet)
% which object is the closest?

[mini, index] = min(distance);
if mini == TISMaxRange(1)
    index = TISdet(1);
end

end

== matlab function ACC_speed_change_curve_cs/Audi_A8_1/PathFollower_1/CTRL REFERENCES/Find Reference Point (pref) on Trajectory closest to PVP Point (pvp)/eml_find_closest_trajectory_points ==
  data: pref output; Actor_traj_distance output; Actor_traj_angle output; pvp input; TrajOffset_x_y_Y input size=3; ActorOffset_Left_Right input; p0 input size=3; Traj_x parameter; Traj_y parameter
function [pref,Actor_traj_distance,Actor_traj_angle]  = eml_find_closest_trajectory_points(pvp,TrajOffset_x_y_Y,ActorOffset_Left_Right,p0,Traj_x,Traj_y)

[pref,Actor_traj_distance,Actor_traj_angle] = emlfcn_find_closest_trajectory_points(pvp,TrajOffset_x_y_Y,ActorOffset_Left_Right,p0,Traj_x,Traj_y,1);

end % end function

== matlab function ACC_speed_change_curve_cs/Audi_A8_1/PathFollower_1/DELTA CTRL/Calculate preview angle/eml_preview_angle_and_distance ==
  data: pvp input; alpha output; pref input; p0 input
function alpha = eml_preview_angle_and_distance(pvp, pref, p0)
%#eml

alpha = emlfcn_preview_angle_and_distance(pvp, pref, p0);

% end function

== matlab function ACC_speed_change_curve_cs/Audi_A8_1/ACC_System3/TIS2 Bend Road/TIS2_closest_object_search1 ==
  data: TISMaxRange parameter; distance input; index output; TISdet parameter
function index = clsst_bjct(TISMaxRange, distance, TISdet)
% which object is the closest?

[mini, index] = min(distance);
if mini == 5*TISMaxRange(2)
    index = TISdet(2);
end
end

== matlab function ACC_speed_change_curve_cs/Audi_A8_1/ACC_System3/TIS2 Straight Road/TIS2_closest_object_search ==
  data: distance input; index output; TISMaxRange parameter; TISdet parameter
function index = clsst_bjct(distance, TISMaxRange, TISdet)
% which object is the closest?

[mini, index] = min(distance);
if mini == 5*TISMaxRange(2)
    index = TISdet(2);
end
end
